simulink model "parte72"  (R2014a)
settings: Solver=ode45  StartTime=0.0  StopTime=10.0  RelTol=1e-3
values from neighbouring files (symbols this model uses):
  z = 0.060    (= 0.06)    [parte72m.m]    (also in parte73_2.m = [0.05 0.01 0.06 ])
settings Model: Creator=Asus  LastModifiedBy=Asus

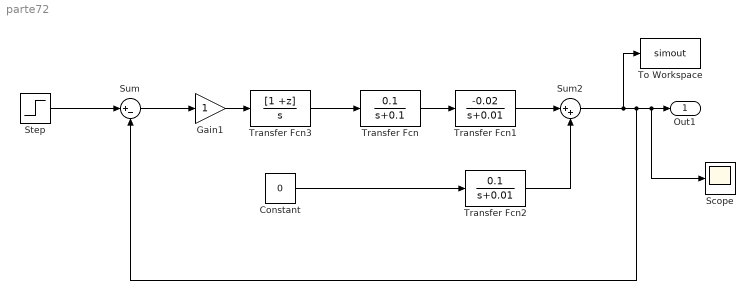
== system parte72 ==
  Constant : Constant  Value=0
  Gain1 : Gain
  Scope : Scope
  Step : Step  SampleTime=0
  Sum : Sum  Inputs=|+-
  Sum2 : Sum  Inputs=|++
  To Workspace : ToWorkspace  VariableName=simout  SaveFormat=Timeseries  SampleTime=-1
  Transfer Fcn : TransferFcn  Numerator=[0.1]  Denominator=[1 0.1]
  Transfer Fcn1 : TransferFcn  Numerator=[-0.02]  Denominator=[1 0.01]
  Transfer Fcn2 : TransferFcn  Numerator=[0.1]  Denominator=[1 0.01]
  Transfer Fcn3 : TransferFcn  Numerator=[1 +z]  Denominator=[1 0]
  Out1 : Outport
  wires:
  Step/1 -> Sum/1
  Transfer Fcn/1 -> Transfer Fcn1/1
  Sum2/1 -> To Workspace/1, Sum/2, Scope/1, Out1/1
  Transfer Fcn1/1 -> Sum2/1
  Transfer Fcn2/1 -> Sum2/2
  Sum/1 -> Gain1/1
  Constant/1 -> Transfer Fcn2/1
  Gain1/1 -> Transfer Fcn3/1
  Transfer Fcn3/1 -> Transfer Fcn/1
